simulink model "sensorMAP"  (R2023a)
settings: Solver=VariableStepAuto  StartTime=0.0  StopTime=10.0  RelTol=1e-3
settings Model: Creator=rafael  LastModifiedBy=rafael

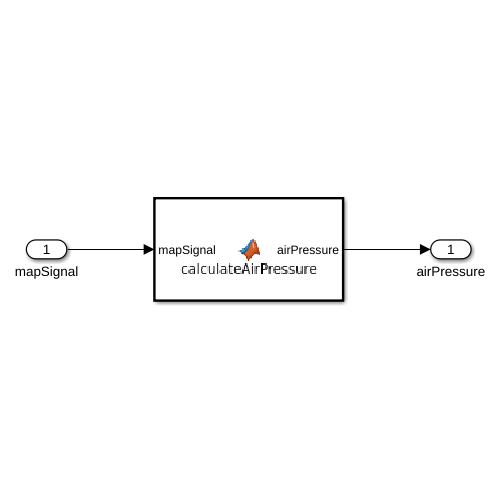
[thumbnail: Simulink's stored preview of the top-level diagram]
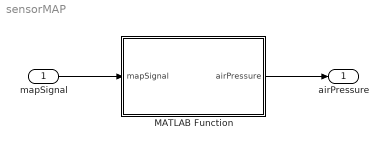
== system sensorMAP ==
  mapSignal : Inport
  MATLAB Function : MATLAB Function  TreatAsAtomicUnit=on
  airPressure : Outport
  wires:
  mapSignal/1 -> MATLAB Function/1(mapSignal)
  MATLAB Function/1(airPressure) -> airPressure/1

== matlab function sensorMAP/MATLAB Function ==
  data: mapSignal input; airPressure output
function airPressure = calculateAirPressure(mapSignal)
    % FUNCTION Calculate Air Pressure
    airPressure = ((0.0435 * mapSignal) + 1.08)*10; 
end
